simulink model "PID_Simulation_System_Discrete_AutoTune"  (R2018b)
settings: Solver=VariableStepAuto  StartTime=0.0  StopTime=6  RelTol=1e-3
undefined symbols (not defined in the file): B, b, g, h, initial_theta, J, Kb, Km, l, La, M, m, max_torque, N, r, Ra
libraries: simulink x2, simulink_extras x1
settings Model: Creator=fred  LastModifiedBy=fredericovaz
settings SolverCC: AlgebraicLoopSolver=LineSearch
settings HardwareCC: ProdBitPerLong=64  ProdHWDeviceType=Intel->x86-64 (Linux 64)

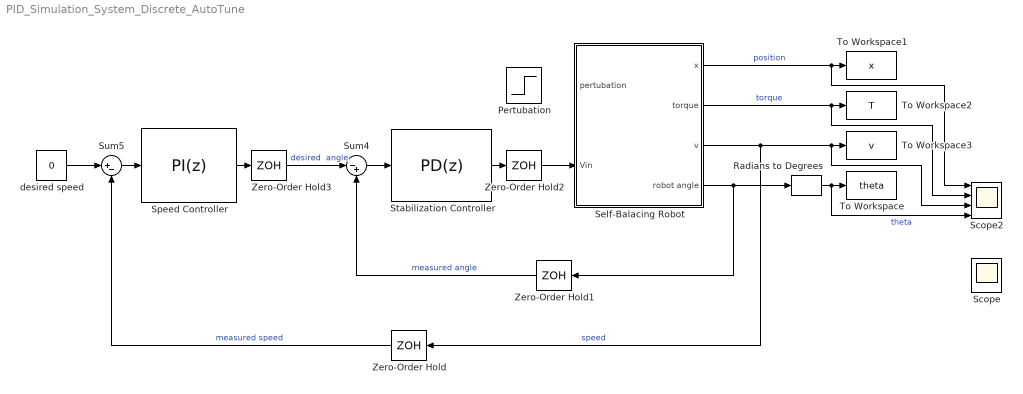
== system PID_Simulation_System_Discrete_AutoTune ==
  Pertubation : Step  Time=7  Before=deg2rad(-1)  After=0  SampleTime=h
  Radians to Degrees : simulink_extras/Transformations/Radians to Degrees
  Scope : Scope
  Scope2 : Scope  NumInputPorts=4
  Self-Balacing Robot : Subsystem
  Speed Controller : simulink/Continuous/PID Controller  Controller=PI  Form=Parallel  TimeDomain=Discrete-time  SampleTime=h  IntegratorMethod=Forward Euler  FilterMethod=Forward Euler  ControllerParametersSource=internal  P=0.107842223159323  I=0.0712804465476108  D=0.00723976610687924  UseFilter=on  N=2285.65595208321  TunerSelectOption=Transfer Function Based (PID Tuner App)  InitialConditionSource=internal  InitialConditionForIntegrator=0  InitialConditionForFilter=0  DifferentiatorICPrevScaledInput=0  ExternalReset=none  TrackingMode=off  Kt=1  LimitOutput=off  UpperSaturationLimit=inf  LowerSaturationLimit=-inf  LinearizeAsGain=on  AntiWindupMode=none  Kb=1  POutMin=[]  POutMax=[]  IOutMin=[]  IOutMax=[]  DOutMin=[]  DOutMax=[]  NOutMin=[]  NOutMax=[]  SumOutMin=[]  SumOutMax=[]  SaturationOutMin=[]  SaturationOutMax=[]  PParamMin=[]  PParamMax=[]  IParamMin=[]  IParamMax=[]  DParamMin=[]  DParamMax=[]  NParamMin=[]  NParamMax=[]  KbParamMin=[]  KbParamMax=[]  KtParamMin=[]  KtParamMax=[]  KbOutMin=[]  KbOutMax=[]  KtOutMin=[]  KtOutMax=[]  IntegratorOutMin=[]  IntegratorOutMax=[]  FilterOutMin=[]  FilterOutMax=[]  SumI1OutMin=[]  SumI1OutMax=[]  SumI2OutMin=[]  SumI2OutMax=[]  SumI3OutMin=[]  SumI3OutMax=[]  SumI4OutMin=[]  SumI4OutMax=[]  SumDOutMin=[]  SumDOutMax=[]  DifferentiatorOutMin=[]  DifferentiatorOutMax=[]  FilterDiffOutCoefMin=[]  FilterDiffOutCoefMax=[]  ReciprocalOutMin=[]  ReciprocalOutMax=[]  SumDenOutMin=[]  SumDenOutMax=[]  SumNumOutMin=[]  SumNumOutMax=[]  DivideOutMin=[]  DivideOutMax=[]  IntegratorContinuousStateAttributes=''  IntegratorStateMustResolveToSignalObject=off  IntegratorRTWStateStorageClass=Auto  FilterContinuousStateAttributes=''  FilterStateMustResolveToSignalObject=off  FilterRTWStateStorageClass=Auto  ParallelPVariant=InternalParameters  IdealPVariant=Disabled  IVariant=InternalParameters  DVariant=Disabled  IntegratorVariant=Discrete  SatVariant=Disabled  AWVariant=Passthrough  PCopyVariant=Disabled  TRVariant=Disabled  FdbkBlocksVariant=Forward  IdealPFdbkVariant=Disabled  SatFdbkVariant=Disabled  DerivativeFilterVariant=Disabled  NVariant=Disabled  NCopyVariant=Disabled_SignalSpec  FilterICVariant=Disabled  IntegratorICVariant=InternalICs  ExternalResetVariant=Disabled  TRSumVariant=Passthrough  SumFdbkVariant=Disabled  SumVariant=Sum_PI
  Stabilization Controller : simulink/Continuous/PID Controller  Controller=PD  Form=Parallel  TimeDomain=Discrete-time  SampleTime=h  IntegratorMethod=Forward Euler  FilterMethod=Forward Euler  ControllerParametersSource=internal  P=49.0772757874348  I=0  D=5.1221003466212  UseFilter=on  N=81.0618695459503  TunerSelectOption=Transfer Function Based (PID Tuner App)  InitialConditionSource=internal  InitialConditionForIntegrator=0  InitialConditionForFilter=0  DifferentiatorICPrevScaledInput=0  ExternalReset=none  TrackingMode=off  Kt=1  LimitOutput=off  UpperSaturationLimit=inf  LowerSaturationLimit=-inf  LinearizeAsGain=on  AntiWindupMode=none  Kb=1  POutMin=[]  POutMax=[]  IOutMin=[]  IOutMax=[]  DOutMin=[]  DOutMax=[]  NOutMin=[]  NOutMax=[]  SumOutMin=[]  SumOutMax=[]  SaturationOutMin=[]  SaturationOutMax=[]  PParamMin=[]  PParamMax=[]  IParamMin=[]  IParamMax=[]  DParamMin=[]  DParamMax=[]  NParamMin=[]  NParamMax=[]  KbParamMin=[]  KbParamMax=[]  KtParamMin=[]  KtParamMax=[]  KbOutMin=[]  KbOutMax=[]  KtOutMin=[]  KtOutMax=[]  IntegratorOutMin=[]  IntegratorOutMax=[]  FilterOutMin=[]  FilterOutMax=[]  SumI1OutMin=[]  SumI1OutMax=[]  SumI2OutMin=[]  SumI2OutMax=[]  SumI3OutMin=[]  SumI3OutMax=[]  SumI4OutMin=[]  SumI4OutMax=[]  SumDOutMin=[]  SumDOutMax=[]  DifferentiatorOutMin=[]  DifferentiatorOutMax=[]  FilterDiffOutCoefMin=[]  FilterDiffOutCoefMax=[]  ReciprocalOutMin=[]  ReciprocalOutMax=[]  SumDenOutMin=[]  SumDenOutMax=[]  SumNumOutMin=[]  SumNumOutMax=[]  DivideOutMin=[]  DivideOutMax=[]  IntegratorContinuousStateAttributes=''  IntegratorStateMustResolveToSignalObject=off  IntegratorRTWStateStorageClass=Auto  FilterContinuousStateAttributes=''  FilterStateMustResolveToSignalObject=off  FilterRTWStateStorageClass=Auto  ParallelPVariant=InternalParameters  IdealPVariant=Disabled  IVariant=Disabled  DVariant=InternalParameters  IntegratorVariant=Disabled  SatVariant=Disabled  AWVariant=Disabled  PCopyVariant=Disabled  TRVariant=Disabled  FdbkBlocksVariant=Forward  IdealPFdbkVariant=Disabled  SatFdbkVariant=Disabled  DerivativeFilterVariant=ForwardEulerFilter  NVariant=InternalParameters  NCopyVariant=Disabled  FilterICVariant=InternalICsFilter  IntegratorICVariant=Disabled  ExternalResetVariant=Disabled  TRSumVariant=Passthrough  SumFdbkVariant=Disabled  SumVariant=Sum_PD
  Sum4 : Sum  Inputs=|-+
  Sum5 : Sum  Inputs=|+-
  To Workspace : ToWorkspace  VariableName=theta  SaveFormat=Timeseries  SampleTime=-1
      settings: Save2DSignal=2-D array (concatenate along first dimension)
  To Workspace1 : ToWorkspace  VariableName=x  SaveFormat=Timeseries  SampleTime=-1
      settings: Save2DSignal=2-D array (concatenate along first dimension)
  To Workspace2 : ToWorkspace  VariableName=T  SaveFormat=Timeseries  SampleTime=-1
      settings: Save2DSignal=2-D array (concatenate along first dimension)
  To Workspace3 : ToWorkspace  VariableName=v  SaveFormat=Timeseries  SampleTime=-1
      settings: Save2DSignal=2-D array (concatenate along first dimension)
  Zero-Order Hold{,1..3} (4 alike) : ZeroOrderHold  SampleTime=h
  desired speed : Constant  Value=0  SampleTime=h
  wires:
  Self-Balacing Robot/4(robot angle) -> Zero-Order Hold1/1, Radians to Degrees/1
  Sum5/1 -> Speed Controller/1
  Stabilization Controller/1 -> Zero-Order Hold2/1
  desired speed/1 -> Sum5/1
  Self-Balacing Robot/3(v) -> Scope2/3, To Workspace3/1, Zero-Order Hold/1  "speed"
  Sum4/1 -> Stabilization Controller/1
  Speed Controller/1 -> Zero-Order Hold3/1
  Zero-Order Hold1/1 -> Sum4/2  "measured angle"
  Zero-Order Hold/1 -> Sum5/2  "measured speed"
  Zero-Order Hold2/1 -> Self-Balacing Robot/2(Vin)
  Self-Balacing Robot/1(x) -> Scope2/1, To Workspace1/1  "position"
  Zero-Order Hold3/1 -> Sum4/1  "desired  angle"
  Radians to Degrees/1 -> Scope2/4, To Workspace/1  "theta"
  Self-Balacing Robot/2(torque) -> Scope2/2, To Workspace2/1  "torque"

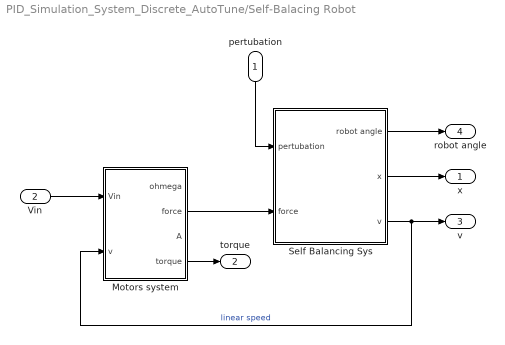
== system PID_Simulation_System_Discrete_AutoTune/Self-Balacing Robot ==
  pertubation : Inport
  Vin : Inport  Port=2
  Motors system : Subsystem
  Self Balancing Sys : Subsystem
  x : Outport
  torque : Outport  Port=2
  v : Outport  Port=3
  robot angle : Outport  Port=4
  wires:
  Self Balancing Sys/1(robot angle) -> robot angle/1
  Self Balancing Sys/3(v) -> Motors system/2(v), v/1  "linear speed"
  Motors system/2(force) -> Self Balancing Sys/2(force)
  Self Balancing Sys/2(x) -> x/1
  Vin/1 -> Motors system/1(Vin)
  pertubation/1 -> Self Balancing Sys/1(pertubation)
  Motors system/4(torque) -> torque/1

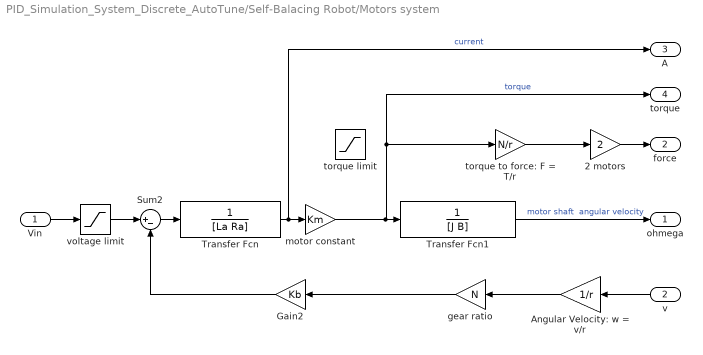
== system PID_Simulation_System_Discrete_AutoTune/Self-Balacing Robot/Motors system ==
  Vin : Inport
  v : Inport  Port=2
  2 motors : Gain  Gain=2
  Angular Velocity: w = v/r : Gain  Gain=1/r
  Gain2 : Gain  Gain=Kb
  Sum2 : Sum  Inputs=|+-
  Transfer Fcn : TransferFcn  Denominator=[La Ra]
  Transfer Fcn1 : TransferFcn  Denominator=[J B]
  gear ratio : Gain  Gain=N
  motor constant : Gain  Gain=Km
  torque limit : Saturate  UpperLimit=max_torque  LowerLimit=-max_torque
  torque to force: F = T/r : Gain  Gain=N/r
  voltage limit : Saturate  UpperLimit=12  LowerLimit=-12
  ohmega : Outport
  force : Outport  Port=2
  A : Outport  Port=3
  torque : Outport  Port=4
  wires:
  Angular Velocity: w = v/r/1 -> gear ratio/1
  motor constant/1 -> torque/1, torque to force: F = T/r/1, Transfer Fcn1/1  "torque"
  Transfer Fcn/1 -> A/1, motor constant/1  "current"
  v/1 -> Angular Velocity: w = v/r/1
  Gain2/1 -> Sum2/2
  Vin/1 -> voltage limit/1
  Sum2/1 -> Transfer Fcn/1
  gear ratio/1 -> Gain2/1
  Transfer Fcn1/1 -> ohmega/1  "motor shaft  angular velocity"
  torque to force: F = T/r/1 -> 2 motors/1
  2 motors/1 -> force/1
  voltage limit/1 -> Sum2/1

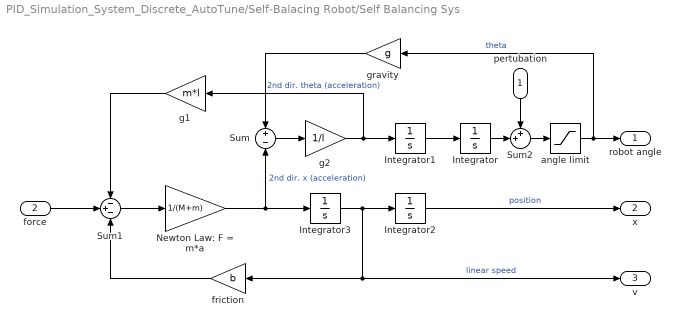
== system PID_Simulation_System_Discrete_AutoTune/Self-Balacing Robot/Self Balancing Sys ==
  pertubation : Inport
  force : Inport  Port=2
  Integrator : Integrator  InitialCondition=initial_theta
  Integrator1 : Integrator
  Integrator2 : Integrator
  Integrator3 : Integrator
  Newton Law: F = m*a : Gain  Gain=1/(M+m)
  Sum : Sum  Inputs=+-
  Sum1 : Sum  Inputs=-+-
  Sum2 : Sum  Inputs=++|
  angle limit : Saturate  UpperLimit=pi/2  LowerLimit=-pi/2
  friction : Gain  Gain=b
  g1 : Gain  Gain=m*l
  g2 : Gain  Gain=1/l
  gravity : Gain  Gain=g
  robot angle : Outport
  x : Outport  Port=2
  v : Outport  Port=3
  wires:
  Sum/1 -> g2/1
  Sum2/1 -> angle limit/1
  Integrator1/1 -> Integrator/1
  force/1 -> Sum1/2
  Integrator/1 -> Sum2/2
  gravity/1 -> Sum/1
  friction/1 -> Sum1/3
  Sum1/1 -> Newton Law: F = m*a/1
  Integrator2/1 -> x/1  "position"
  Newton Law: F = m*a/1 -> Sum/2, Integrator3/1  "2nd dir. x (acceleration)"
  g1/1 -> Sum1/1
  Integrator3/1 -> v/1, friction/1, Integrator2/1  "linear speed"
  g2/1 -> g1/1, Integrator1/1  "2nd dir. theta (acceleration)"
  pertubation/1 -> Sum2/1
  angle limit/1 -> gravity/1, robot angle/1  "theta"
